simulink model "Atest"  (R2021a)
settings: Solver=VariableStepAuto  StartTime=0.0  StopTime=10.0  RelTol=1e-3
model workspace: external: MAT-File params.mat (data not in the file)
settings Model: OrderedModelArguments=off  Creator=johna  LastModifiedBy=johna

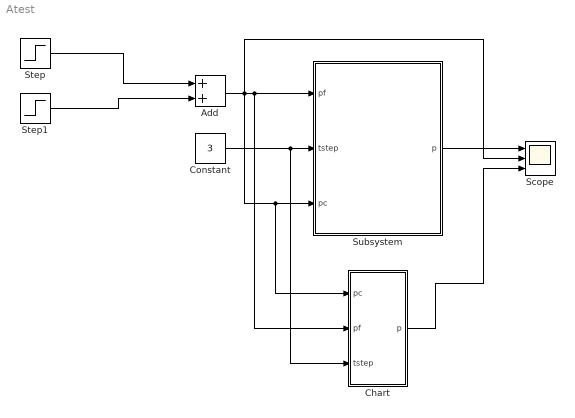
== system Atest ==
  Add : Sum
  Chart : Stateflow chart  TreatAsAtomicUnit=on
  Constant : Constant  Value=3
  Scope : Scope  NumInputPorts=3
  Step : Step  Time=5  Before=8  After=-8
  Step1 : Step  Time=3  Before=-5  After=6  SampleTime=0
  Subsystem : Subsystem
  wires:
  Step/1 -> Add/1
  Constant/1 -> Chart/3(tstep), Subsystem/2(tstep)
  Subsystem/1(p) -> Scope/1
  Step1/1 -> Add/2
  Add/1 -> Chart/1(pc), Subsystem/3(pc), Chart/2(pf), Subsystem/1(pf), Scope/2
  Chart/1(p) -> Scope/3

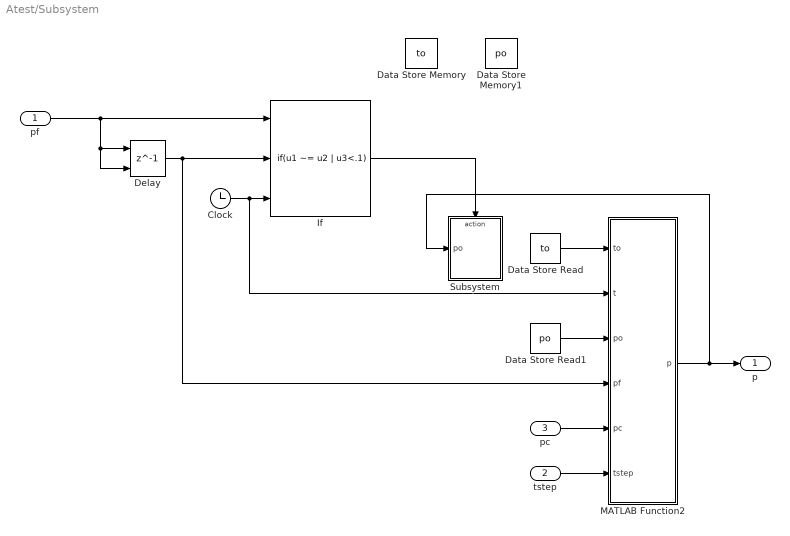
== system Atest/Subsystem ==
  pf : Inport
  tstep : Inport  Port=2
  pc : Inport  Port=3
  Clock : Clock
  Data Store Memory : DataStoreMemory  DataStoreName=to  ReadBeforeWriteMsg=warning  WriteAfterWriteMsg=warning  WriteAfterReadMsg=warning  ShowAdditionalParam=off
  Data Store Memory1 : DataStoreMemory  DataStoreName=po  ReadBeforeWriteMsg=warning  WriteAfterWriteMsg=warning  WriteAfterReadMsg=warning  ShowAdditionalParam=off
  Data Store Read : DataStoreRead  DataStoreName=to  IndexOptions=Index vector (dialog)  Indices=1  OutputSizes=1
  Data Store Read1 : DataStoreRead  DataStoreName=po  IndexOptions=Index vector (dialog)  Indices=1  OutputSizes=1
  Delay : Delay  DelayLength=1  InitialConditionSource=Input port
      settings: InputPortMap=u0,p4
  If : If  NumInputs=3  IfExpression=u1 ~= u2 | u3<.1  ShowElse=off
  MATLAB Function2 : MATLAB Function  TreatAsAtomicUnit=on
  Subsystem : Subsystem
  p : Outport
  wires:
  Clock/1 -> MATLAB Function2/2(t), If/3
  MATLAB Function2/1(p) -> Subsystem/1(po), p/1
  tstep/1 -> MATLAB Function2/6(tstep)
  pf/1 -> Delay/2, Delay/1, If/1
  If/1 -> Subsystem/Action
  Delay/1 -> MATLAB Function2/4(pf), If/2
  Data Store Read/1 -> MATLAB Function2/1(to)
  Data Store Read1/1 -> MATLAB Function2/3(po)
  pc/1 -> MATLAB Function2/5(pc)

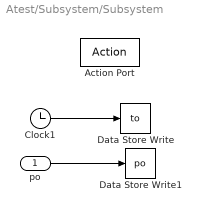
== system Atest/Subsystem/Subsystem ==
  po : Inport
  Action Port : ActionPort  ActionPortLabel=if(u1 ~= u2 | u3<.1)
  Clock1 : Clock
  Data Store Write : DataStoreWrite  DataStoreName=to  IndexOptions=Index vector (dialog)  Indices=1  OutputSizes=1
  Data Store Write1 : DataStoreWrite  DataStoreName=po  IndexOptions=Index vector (dialog)  Indices=1  OutputSizes=1
  wires:
  Clock1/1 -> Data Store Write/1
  po/1 -> Data Store Write1/1

== stateflow chart Atest/Chart ==
  state Ramp
    entry:
    to = t
    ptemp = pf;
    po = p;
    slope = (pf - po)/tstep
    during:
    p = po + slope*(t-to);
  state Ideal
  (default) -> Ramp : {p = pc;
      | ptemp = pf;}
  Ideal -> Ramp : [ptemp~=pf]
  Ramp -> Ramp [order 1] : [ptemp~=pf]
  Ramp -> Ideal [order 2] : [(p >= pf & slope>0) | (p <= pf & slope<0)]
      | {p = pf;}
  data: pc input; pf input; tstep input; po local; slope local; to local; p output; ptemp local

== matlab function Atest/Subsystem/MATLAB Function2 ==
  data: to input; p output; t input; po input; pf input; pc input; tstep input
function p = ramp(to,t,po,pf,pc, tstep)
    slope = (pf - po)/tstep;
    p = po + slope*(t-to);
    if((p > pf&& slope>0) || (p < pf && slope<0))
        p = pf;
    end
    if(t==0)
        p = pc;
    end
